simulink model "Non_linear_sloshing"  (R2024a)
settings: Solver=ode4  StartTime=0.0  StopTime=100  FixedStep=0.01  RelTol=1e-3
values from neighbouring files (symbols this model uses):
  damping = 0.003    [Non_linear_sloshing.m]
  pendulums = sloshing_pendulums(params, 4)    [Non_linear_sloshing.m]
settings Model: Creator=Pinoi  LastModifiedBy=Pinoi
settings OptimizationCC: BlockReduction=off  DefaultParameterBehavior=Inlined  BufferReuse=off

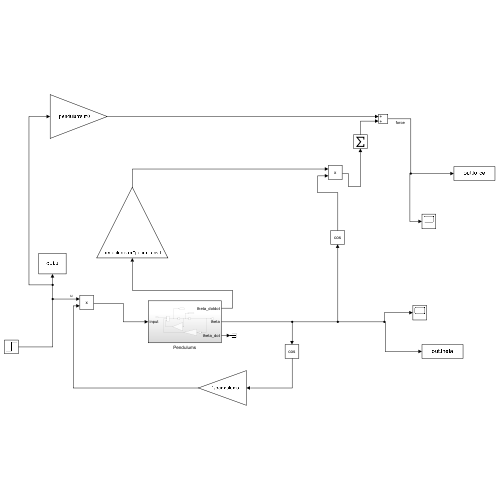
[thumbnail: Simulink's stored preview of the top-level diagram]
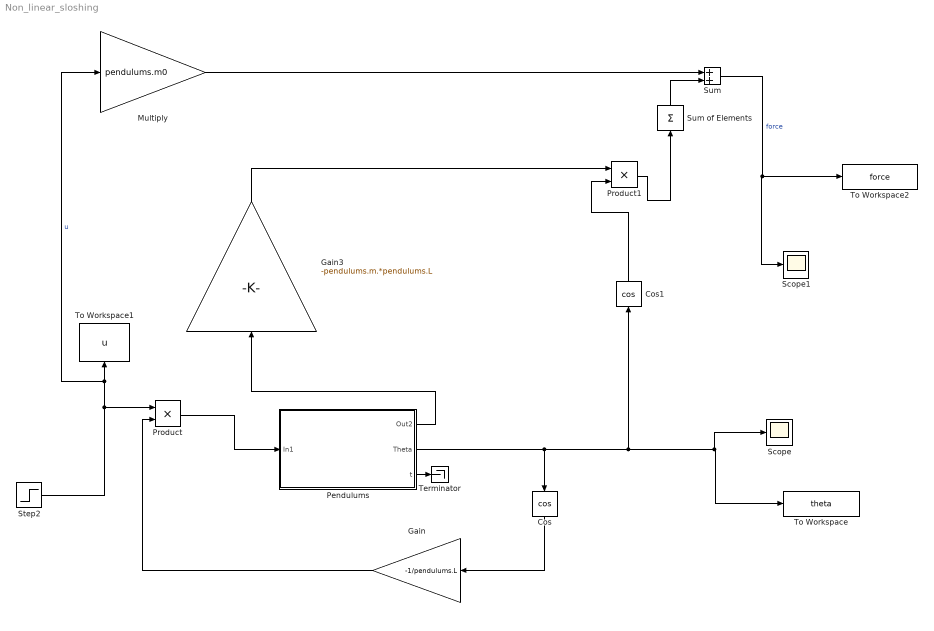
== system Non_linear_sloshing ==
  Cos : Trigonometry  Operator=cos
  Cos1 : Trigonometry  Operator=cos
  Gain : Gain  Gain=-1/pendulums.L
  Gain3 : Gain  Gain=-pendulums.m.*pendulums.L
  Multiply : Gain  Gain=pendulums.m0
  Pendulums : Subsystem
  Product : Product
  Product1 : Product
  Scope : Scope
  Scope1 : Scope
  Step2 : Step  Time=0  SampleTime=0
  Sum : Sum
  Sum of Elements : Sum  Inputs=+
  Terminator : Terminator
  To Workspace : ToWorkspace  VariableName=theta  SampleTime=-1
  To Workspace1 : ToWorkspace  VariableName=u  SampleTime=-1
  To Workspace2 : ToWorkspace  VariableName=force  SampleTime=-1
      settings: Save2DSignal=2-D array (concatenate along first dimension)
  wires:
  Step2/1 -> Multiply/1, To Workspace1/1, Product/1  "u"
  Gain/1 -> Product/2
  Cos/1 -> Gain/1
  Gain3/1 -> Product1/1
  Cos1/1 -> Product1/2
  Multiply/1 -> Sum/1
  Sum/1 -> Scope1/1, To Workspace2/1  "force"
  Product/1 -> Pendulums/1(In1)
  Pendulums/2(Theta) -> Cos1/1, Scope/1, To Workspace/1, Cos/1
  Pendulums/1(Out2) -> Gain3/1
  Pendulums/3(t) -> Terminator/1
  Sum of Elements/1 -> Sum/2
  Product1/1 -> Sum of Elements/1

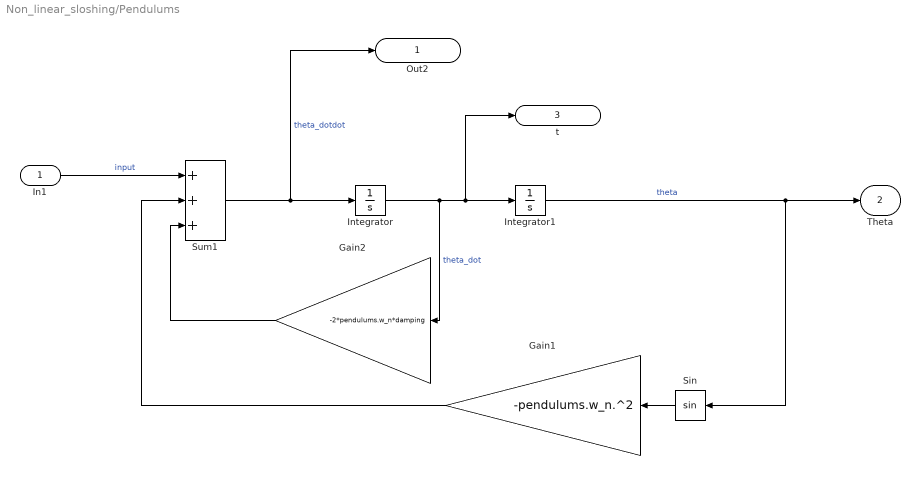
== system Non_linear_sloshing/Pendulums ==
  In1 : Inport
  Gain1 : Gain  Gain=-pendulums.w_n.^2
  Gain2 : Gain  Gain=-2*pendulums.w_n*damping
  Integrator : Integrator
  Integrator1 : Integrator
  Sin : Trigonometry
  Sum1 : Sum  Inputs=+++
  Out2 : Outport
  Theta : Outport  Port=2
  t : Outport  Port=3
  wires:
  Gain1/1 -> Sum1/2
  Gain2/1 -> Sum1/3
  Integrator1/1 -> Sin/1, Theta/1  "theta"
  Sin/1 -> Gain1/1
  Sum1/1 -> Out2/1, Integrator/1  "theta_dotdot"
  Integrator/1 -> Gain2/1, t/1, Integrator1/1  "theta_dot"
  In1/1 -> Sum1/1  "input"
